simulink model "sampleModel7127_pp_difftest"  (R2018a)
settings: Solver=VariableStepAuto  StartTime=0.0  StopTime=10.0  RelTol=1e-3
undefined symbols (not defined in the file or in its folder): DiscIntNeverNeededParam, sigbuilder_block
libraries: simulink x258
(part 2 of 5)

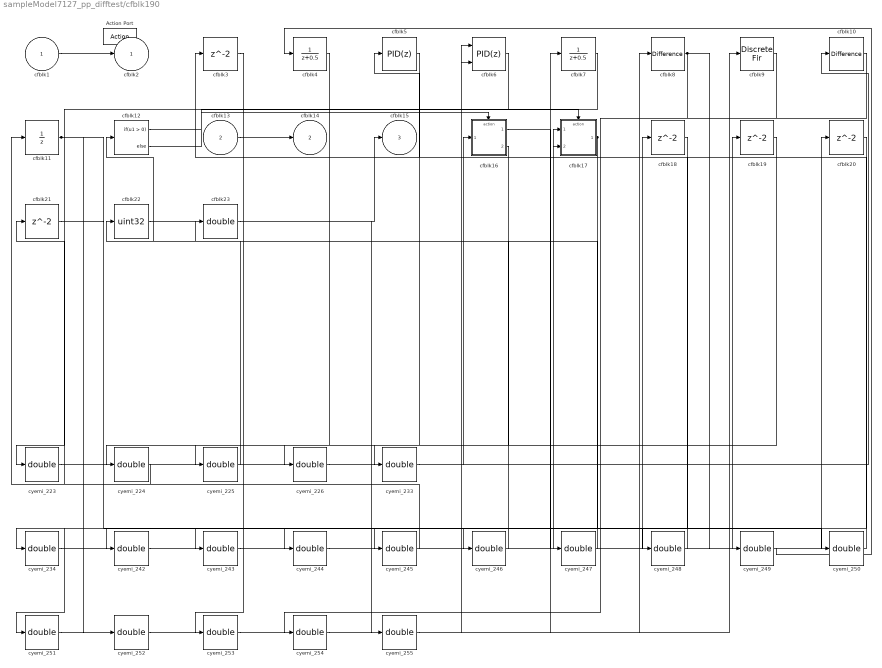
== system sampleModel7127_pp_difftest/cfblk190 ==
  cfblk1 : Inport
  cfblk13 : Inport  Port=2
  Action Port : ActionPort  ActionType=else
  cfblk10 : simulink/Discrete/Difference  ICPrevInput=0.0  OutMin=[]  OutMax=[]  OutDataTypeStr=double  OutputDataTypeScalingMode=double  OutDataType=fixdt(1, 16)  OutScaling=2^-10  DoSatur=off
  cfblk11 : UnitDelay  SampleTime=-1
  cfblk12 : If  SampleTime=1
  cfblk16 : Subsystem  TreatAsAtomicUnit=on
  cfblk17 : Subsystem  TreatAsAtomicUnit=on
  cfblk{3,18..21} (5 alike) : Delay
  cfblk22 : DataTypeConversion  OutDataTypeStr=uint32
  cfblk23 : DataTypeConversion  OutDataTypeStr=double
  cfblk4 : DiscreteTransferFcn
  cfblk5 : simulink/Continuous/PID Controller  Controller=PID  TimeDomain=Discrete-time  SampleTime=-1  IntegratorMethod=Forward Euler  FilterMethod=Forward Euler  Form=Parallel  UseFilter=on  ControllerParametersSource=internal  P=1  I=1  D=0  N=100  InitialConditionSource=internal  InitialConditionForIntegrator=0  InitialConditionForFilter=0  ExternalReset=none  LimitOutput=off  UpperSaturationLimit=inf  LowerSaturationLimit=-inf  LinearizeAsGain=off  AntiWindupMode=none  Kb=1  TrackingMode=off  Kt=1  PParamMin=[]  PParamMax=[]  IParamMin=[]  IParamMax=[]  DParamMin=[]  DParamMax=[]  NParamMin=[]  NParamMax=[]  KbParamMin=[]  KbParamMax=[]  KtParamMin=[]  KtParamMax=[]  POutMin=[]  POutMax=[]  IOutMin=[]  IOutMax=[]  DOutMin=[]  DOutMax=[]  NOutMin=[]  NOutMax=[]  KbOutMin=[]  KbOutMax=[]  KtOutMin=[]  KtOutMax=[]  IntegratorOutMin=[]  IntegratorOutMax=[]  FilterOutMin=[]  FilterOutMax=[]  SumOutMin=[]  SumOutMax=[]  SumI1OutMin=[]  SumI1OutMax=[]  SumI2OutMin=[]  SumI2OutMax=[]  SumI3OutMin=[]  SumI3OutMax=[]  SumDOutMin=[]  SumDOutMax=[]  SaturationOutMin=[]  SaturationOutMax=[]  IntegratorContinuousStateAttributes=''  IntegratorStateMustResolveToSignalObject=off  IntegratorRTWStateStorageClass=Auto  FilterContinuousStateAttributes=''  FilterStateMustResolveToSignalObject=off  FilterRTWStateStorageClass=Auto  DifferentiatorICPrevScaledInput=0  DifferentiatorOutMin=[]  DifferentiatorOutMax=[]  FilterDiffOutCoefMin=[]  FilterDiffOutCoefMax=[]  SumDenOutMin=[]  SumDenOutMax=[]  SumNumOutMin=[]  SumNumOutMax=[]  ReciprocalOutMin=[]  ReciprocalOutMax=[]  DivideOutMin=[]  DivideOutMax=[]  TunerSelectOption=Transfer Function Based (PID Tuner App)
  cfblk6 : simulink/Continuous/PID Controller (2DOF)  Controller=PID  TimeDomain=Discrete-time  SampleTime=-1  IntegratorMethod=Forward Euler  FilterMethod=Forward Euler  Form=Parallel  UseFilter=on  ControllerParametersSource=internal  P=1  I=1  D=0  N=100  b=1  c=1  InitialConditionSource=internal  InitialConditionForIntegrator=0  InitialConditionForFilter=0  ExternalReset=none  LimitOutput=off  UpperSaturationLimit=inf  LowerSaturationLimit=-inf  LinearizeAsGain=off  AntiWindupMode=none  Kb=1  TrackingMode=off  Kt=1  PParamMin=[]  PParamMax=[]  IParamMin=[]  IParamMax=[]  DParamMin=[]  DParamMax=[]  NParamMin=[]  NParamMax=[]  bParamMin=[]  bParamMax=[]  cParamMin=[]  cParamMax=[]  KbParamMin=[]  KbParamMax=[]  KtParamMin=[]  KtParamMax=[]  POutMin=[]  POutMax=[]  IOutMin=[]  IOutMax=[]  DOutMin=[]  DOutMax=[]  NOutMin=[]  NOutMax=[]  bOutMin=[]  bOutMax=[]  cOutMin=[]  cOutMax=[]  KbOutMin=[]  KbOutMax=[]  KtOutMin=[]  KtOutMax=[]  IntegratorOutMin=[]  IntegratorOutMax=[]  FilterOutMin=[]  FilterOutMax=[]  SumOutMin=[]  SumOutMax=[]  Sum1OutMin=[]  Sum1OutMax=[]  Sum2OutMin=[]  Sum2OutMax=[]  Sum3OutMin=[]  Sum3OutMax=[]  SumI1OutMin=[]  SumI1OutMax=[]  SumI2OutMin=[]  SumI2OutMax=[]  SumI3OutMin=[]  SumI3OutMax=[]  SumDOutMin=[]  SumDOutMax=[]  SaturationOutMin=[]  SaturationOutMax=[]  IntegratorContinuousStateAttributes=''  IntegratorStateMustResolveToSignalObject=off  IntegratorRTWStateStorageClass=Auto  FilterContinuousStateAttributes=''  FilterStateMustResolveToSignalObject=off  FilterRTWStateStorageClass=Auto  DifferentiatorICPrevScaledInput=0  DifferentiatorOutMin=[]  DifferentiatorOutMax=[]  FilterDiffOutCoefMin=[]  FilterDiffOutCoefMax=[]  SumDenOutMin=[]  SumDenOutMax=[]  SumNumOutMin=[]  SumNumOutMax=[]  ReciprocalOutMin=[]  ReciprocalOutMax=[]  DivideOutMin=[]  DivideOutMax=[]  TunerSelectOption=Transfer Function Based (PID Tuner App)
  cfblk7 : DiscreteTransferFcn
  cfblk8 : simulink/Discrete/Difference  ICPrevInput=0.0  OutMin=[]  OutMax=[]  OutDataTypeStr=double  OutputDataTypeScalingMode=double  OutDataType=fixdt(1, 16)  OutScaling=2^-10  DoSatur=off
  cfblk9 : DiscreteFir
  cyemi_{223..226,233..234,242..255} (20 alike) : DataTypeConversion  OutDataTypeStr=double
  cfblk2 : Outport
  cfblk14 : Outport  Port=2
  cfblk15 : Outport  Port=3
  wires:
  cfblk13/1 -> cfblk14/1
  cfblk1/1 -> cfblk2/1
  cfblk17/1(cfblk2) -> cyemi_242/1, cyemi_251/1
  cfblk8/1 -> cyemi_244/1, cyemi_249/1
  cfblk11/1 -> cyemi_245/1, cyemi_252/1
  cfblk12/1 -> cfblk16/Action
  cfblk12/2 -> cfblk17/Action
  cfblk22/1 -> cfblk15/1
  cyemi_223/1 -> cfblk10/1
  cfblk6/1 -> cyemi_223/1
  cyemi_224/1 -> cfblk11/1
  cfblk5/1 -> cyemi_224/1
  cyemi_225/1 -> cfblk12/1
  cfblk3/1 -> cyemi_225/1
  cyemi_226/1 -> cfblk16/1(cfblk1)
  cfblk19/1 -> cyemi_226/1
  cyemi_233/1 -> cfblk17/1(cfblk1)
  cfblk16/2(cfblk7) -> cyemi_233/1
  cyemi_234/1 -> cfblk17/2(cfblk9)
  cfblk20/1 -> cyemi_234/1
  cyemi_242/1 -> cfblk18/1
  cyemi_243/1 -> cfblk19/1
  cfblk7/1 -> cyemi_243/1
  cyemi_244/1 -> cfblk20/1
  cyemi_245/1 -> cfblk21/1
  cyemi_246/1 -> cfblk22/1
  cfblk9/1 -> cyemi_246/1
  cyemi_247/1 -> cfblk23/1
  cfblk16/1(cfblk2) -> cyemi_247/1
  cyemi_248/1 -> cfblk3/1
  cfblk18/1 -> cyemi_248/1
  cyemi_249/1 -> cfblk4/1
  cyemi_250/1 -> cfblk5/1
  cfblk21/1 -> cyemi_250/1
  cyemi_251/1 -> cfblk6/1
  cyemi_252/1 -> cfblk6/2
  cyemi_253/1 -> cfblk7/1
  cfblk4/1 -> cyemi_253/1
  cyemi_254/1 -> cfblk8/1
  cfblk10/1 -> cyemi_254/1
  cyemi_255/1 -> cfblk9/1
  cfblk23/1 -> cyemi_255/1

== system sampleModel7127_pp_difftest/cfblk191 ==
  cfblk1 : Inport
  Action Port : ActionPort  ActionType=then
  cfblk10 : DiscreteFir
  cfblk11 : simulink/Continuous/PID Controller  Controller=PID  TimeDomain=Discrete-time  SampleTime=-1  IntegratorMethod=Forward Euler  FilterMethod=Forward Euler  Form=Parallel  UseFilter=on  ControllerParametersSource=internal  P=1  I=1  D=0  N=100  InitialConditionSource=internal  InitialConditionForIntegrator=0  InitialConditionForFilter=0  ExternalReset=none  LimitOutput=off  UpperSaturationLimit=inf  LowerSaturationLimit=-inf  LinearizeAsGain=off  AntiWindupMode=none  Kb=1  TrackingMode=off  Kt=1  PParamMin=[]  PParamMax=[]  IParamMin=[]  IParamMax=[]  DParamMin=[]  DParamMax=[]  NParamMin=[]  NParamMax=[]  KbParamMin=[]  KbParamMax=[]  KtParamMin=[]  KtParamMax=[]  POutMin=[]  POutMax=[]  IOutMin=[]  IOutMax=[]  DOutMin=[]  DOutMax=[]  NOutMin=[]  NOutMax=[]  KbOutMin=[]  KbOutMax=[]  KtOutMin=[]  KtOutMax=[]  IntegratorOutMin=[]  IntegratorOutMax=[]  FilterOutMin=[]  FilterOutMax=[]  SumOutMin=[]  SumOutMax=[]  SumI1OutMin=[]  SumI1OutMax=[]  SumI2OutMin=[]  SumI2OutMax=[]  SumI3OutMin=[]  SumI3OutMax=[]  SumDOutMin=[]  SumDOutMax=[]  SaturationOutMin=[]  SaturationOutMax=[]  IntegratorContinuousStateAttributes=''  IntegratorStateMustResolveToSignalObject=off  IntegratorRTWStateStorageClass=Auto  FilterContinuousStateAttributes=''  FilterStateMustResolveToSignalObject=off  FilterRTWStateStorageClass=Auto  DifferentiatorICPrevScaledInput=0  DifferentiatorOutMin=[]  DifferentiatorOutMax=[]  FilterDiffOutCoefMin=[]  FilterDiffOutCoefMax=[]  SumDenOutMin=[]  SumDenOutMax=[]  SumNumOutMin=[]  SumNumOutMax=[]  ReciprocalOutMin=[]  ReciprocalOutMax=[]  DivideOutMin=[]  DivideOutMax=[]  TunerSelectOption=Transfer Function Based (PID Tuner App)
  cfblk12 : simulink/Continuous/PID Controller  Controller=PID  TimeDomain=Discrete-time  SampleTime=-1  IntegratorMethod=Forward Euler  FilterMethod=Forward Euler  Form=Parallel  UseFilter=on  ControllerParametersSource=internal  P=1  I=1  D=0  N=100  InitialConditionSource=internal  InitialConditionForIntegrator=0  InitialConditionForFilter=0  ExternalReset=none  LimitOutput=off  UpperSaturationLimit=inf  LowerSaturationLimit=-inf  LinearizeAsGain=off  AntiWindupMode=none  Kb=1  TrackingMode=off  Kt=1  PParamMin=[]  PParamMax=[]  IParamMin=[]  IParamMax=[]  DParamMin=[]  DParamMax=[]  NParamMin=[]  NParamMax=[]  KbParamMin=[]  KbParamMax=[]  KtParamMin=[]  KtParamMax=[]  POutMin=[]  POutMax=[]  IOutMin=[]  IOutMax=[]  DOutMin=[]  DOutMax=[]  NOutMin=[]  NOutMax=[]  KbOutMin=[]  KbOutMax=[]  KtOutMin=[]  KtOutMax=[]  IntegratorOutMin=[]  IntegratorOutMax=[]  FilterOutMin=[]  FilterOutMax=[]  SumOutMin=[]  SumOutMax=[]  SumI1OutMin=[]  SumI1OutMax=[]  SumI2OutMin=[]  SumI2OutMax=[]  SumI3OutMin=[]  SumI3OutMax=[]  SumDOutMin=[]  SumDOutMax=[]  SaturationOutMin=[]  SaturationOutMax=[]  IntegratorContinuousStateAttributes=''  IntegratorStateMustResolveToSignalObject=off  IntegratorRTWStateStorageClass=Auto  FilterContinuousStateAttributes=''  FilterStateMustResolveToSignalObject=off  FilterRTWStateStorageClass=Auto  DifferentiatorICPrevScaledInput=0  DifferentiatorOutMin=[]  DifferentiatorOutMax=[]  FilterDiffOutCoefMin=[]  FilterDiffOutCoefMax=[]  SumDenOutMin=[]  SumDenOutMax=[]  SumNumOutMin=[]  SumNumOutMax=[]  ReciprocalOutMin=[]  ReciprocalOutMax=[]  DivideOutMin=[]  DivideOutMax=[]  TunerSelectOption=Transfer Function Based (PID Tuner App)
  cfblk13 : simulink/Discrete/Difference  ICPrevInput=0.0  OutMin=[]  OutMax=[]  OutDataTypeStr=double  OutputDataTypeScalingMode=double  OutDataType=fixdt(1, 16)  OutScaling=2^-10  DoSatur=off
  cfblk14 : Delay
  cfblk15 : Delay
  cfblk3 : simulink/Discrete/Transfer Fcn First Order  PoleZ=0.95  ICPrevOutput=0.0  DoSatur=off
      settings: SourceProductName=Simulink
  cfblk4 : DiscreteZeroPole  Poles=[0 0.5]  Gain=1  SampleTime=-1
  cfblk5 : DiscreteTransferFcn
  cfblk6 : simulink/Continuous/PID Controller  Controller=PID  TimeDomain=Discrete-time  SampleTime=-1  IntegratorMethod=Forward Euler  FilterMethod=Forward Euler  Form=Parallel  UseFilter=on  ControllerParametersSource=internal  P=1  I=1  D=0  N=100  InitialConditionSource=internal  InitialConditionForIntegrator=0  InitialConditionForFilter=0  ExternalReset=none  LimitOutput=off  UpperSaturationLimit=inf  LowerSaturationLimit=-inf  LinearizeAsGain=off  AntiWindupMode=none  Kb=1  TrackingMode=off  Kt=1  PParamMin=[]  PParamMax=[]  IParamMin=[]  IParamMax=[]  DParamMin=[]  DParamMax=[]  NParamMin=[]  NParamMax=[]  KbParamMin=[]  KbParamMax=[]  KtParamMin=[]  KtParamMax=[]  POutMin=[]  POutMax=[]  IOutMin=[]  IOutMax=[]  DOutMin=[]  DOutMax=[]  NOutMin=[]  NOutMax=[]  KbOutMin=[]  KbOutMax=[]  KtOutMin=[]  KtOutMax=[]  IntegratorOutMin=[]  IntegratorOutMax=[]  FilterOutMin=[]  FilterOutMax=[]  SumOutMin=[]  SumOutMax=[]  SumI1OutMin=[]  SumI1OutMax=[]  SumI2OutMin=[]  SumI2OutMax=[]  SumI3OutMin=[]  SumI3OutMax=[]  SumDOutMin=[]  SumDOutMax=[]  SaturationOutMin=[]  SaturationOutMax=[]  IntegratorContinuousStateAttributes=''  IntegratorStateMustResolveToSignalObject=off  IntegratorRTWStateStorageClass=Auto  FilterContinuousStateAttributes=''  FilterStateMustResolveToSignalObject=off  FilterRTWStateStorageClass=Auto  DifferentiatorICPrevScaledInput=0  DifferentiatorOutMin=[]  DifferentiatorOutMax=[]  FilterDiffOutCoefMin=[]  FilterDiffOutCoefMax=[]  SumDenOutMin=[]  SumDenOutMax=[]  SumNumOutMin=[]  SumNumOutMax=[]  ReciprocalOutMin=[]  ReciprocalOutMax=[]  DivideOutMin=[]  DivideOutMax=[]  TunerSelectOption=Transfer Function Based (PID Tuner App)
  cfblk7 : simulink/Discrete/Transfer Fcn Real Zero  ZeroZ=0.75  ICPrevInput=0.0  DoSatur=off
      settings: SourceProductName=Simulink  SourceProductBaseCode=SL
  cfblk8 : simulink/Discrete/Tapped Delay  vinit=0.0  samptime=-1  NumDelays=1  DelayOrder=Oldest  includeCurrent=off
  cfblk9 : simulink/Discrete/Difference  ICPrevInput=0.0  OutMin=[]  OutMax=[]  OutDataTypeStr=double  OutputDataTypeScalingMode=double  OutDataType=fixdt(1, 16)  OutScaling=2^-10  DoSatur=off
  cyemi_{257..269} (13 alike) : DataTypeConversion  OutDataTypeStr=double
  cfblk2 : Outport
  wires:
  cfblk1/1 -> cfblk2/1
  cyemi_257/1 -> cfblk10/1
  cfblk11/1 -> cyemi_257/1
  cyemi_258/1 -> cfblk11/1
  cfblk7/1 -> cyemi_258/1
  cyemi_259/1 -> cfblk12/1
  cfblk3/1 -> cyemi_259/1
  cyemi_260/1 -> cfblk13/1
  cfblk8/1 -> cyemi_260/1
  cyemi_261/1 -> cfblk14/1
  cfblk10/1 -> cyemi_261/1
  cyemi_262/1 -> cfblk15/1
  cfblk9/1 -> cyemi_262/1
  cyemi_263/1 -> cfblk3/1
  cfblk14/1 -> cyemi_263/1
  cyemi_264/1 -> cfblk4/1
  cfblk15/1 -> cyemi_264/1
  cyemi_265/1 -> cfblk5/1
  cfblk13/1 -> cyemi_265/1
  cyemi_266/1 -> cfblk6/1
  cfblk5/1 -> cyemi_266/1
  cyemi_267/1 -> cfblk7/1
  cfblk6/1 -> cyemi_267/1
  cyemi_268/1 -> cfblk8/1
  cfblk12/1 -> cyemi_268/1
  cyemi_269/1 -> cfblk9/1
  cfblk4/1 -> cyemi_269/1

== system sampleModel7127_pp_difftest/cfblk192 ==
  cfblk1 : Inport
  cfblk8 : Inport  Port=2
  Action Port : ActionPort  ActionType=else
  cfblk3 : DiscreteStateSpace  SampleTime=-1
  cfblk4 : simulink/Discrete/Transfer Fcn Real Zero  ZeroZ=0.75  ICPrevInput=0.0  DoSatur=off
      settings: SourceProductName=Simulink  SourceProductBaseCode=SL
  cfblk5 : simulink/Discrete/Difference  ICPrevInput=0.0  OutMin=[]  OutMax=[]  OutDataTypeStr=double  OutputDataTypeScalingMode=double  OutDataType=fixdt(1, 16)  OutScaling=2^-10  DoSatur=off
  cfblk6 : DiscreteZeroPole  Poles=[0 0.5]  Gain=1  SampleTime=-1
  cfblk7 : simulink/Continuous/PID Controller (2DOF)  Controller=PID  TimeDomain=Discrete-time  SampleTime=-1  IntegratorMethod=Forward Euler  FilterMethod=Forward Euler  Form=Parallel  UseFilter=on  ControllerParametersSource=internal  P=1  I=1  D=0  N=100  b=1  c=1  InitialConditionSource=internal  InitialConditionForIntegrator=0  InitialConditionForFilter=0  ExternalReset=none  LimitOutput=off  UpperSaturationLimit=inf  LowerSaturationLimit=-inf  LinearizeAsGain=off  AntiWindupMode=none  Kb=1  TrackingMode=off  Kt=1  PParamMin=[]  PParamMax=[]  IParamMin=[]  IParamMax=[]  DParamMin=[]  DParamMax=[]  NParamMin=[]  NParamMax=[]  bParamMin=[]  bParamMax=[]  cParamMin=[]  cParamMax=[]  KbParamMin=[]  KbParamMax=[]  KtParamMin=[]  KtParamMax=[]  POutMin=[]  POutMax=[]  IOutMin=[]  IOutMax=[]  DOutMin=[]  DOutMax=[]  NOutMin=[]  NOutMax=[]  bOutMin=[]  bOutMax=[]  cOutMin=[]  cOutMax=[]  KbOutMin=[]  KbOutMax=[]  KtOutMin=[]  KtOutMax=[]  IntegratorOutMin=[]  IntegratorOutMax=[]  FilterOutMin=[]  FilterOutMax=[]  SumOutMin=[]  SumOutMax=[]  Sum1OutMin=[]  Sum1OutMax=[]  Sum2OutMin=[]  Sum2OutMax=[]  Sum3OutMin=[]  Sum3OutMax=[]  SumI1OutMin=[]  SumI1OutMax=[]  SumI2OutMin=[]  SumI2OutMax=[]  SumI3OutMin=[]  SumI3OutMax=[]  SumDOutMin=[]  SumDOutMax=[]  SaturationOutMin=[]  SaturationOutMax=[]  IntegratorContinuousStateAttributes=''  IntegratorStateMustResolveToSignalObject=off  IntegratorRTWStateStorageClass=Auto  FilterContinuousStateAttributes=''  FilterStateMustResolveToSignalObject=off  FilterRTWStateStorageClass=Auto  DifferentiatorICPrevScaledInput=0  DifferentiatorOutMin=[]  DifferentiatorOutMax=[]  FilterDiffOutCoefMin=[]  FilterDiffOutCoefMax=[]  SumDenOutMin=[]  SumDenOutMax=[]  SumNumOutMin=[]  SumNumOutMax=[]  ReciprocalOutMin=[]  ReciprocalOutMax=[]  DivideOutMin=[]  DivideOutMax=[]  TunerSelectOption=Transfer Function Based (PID Tuner App)
  cfblk9 : Delay
  cyemi_{272..278} (7 alike) : DataTypeConversion  OutDataTypeStr=double
  cfblk2 : Outport
  wires:
  cfblk1/1 -> cfblk2/1
  cyemi_272/1 -> cfblk3/1
  cfblk9/1 -> cyemi_272/1
  cyemi_273/1 -> cfblk4/1
  cfblk5/1 -> cyemi_273/1
  cyemi_274/1 -> cfblk5/1
  cfblk7/1 -> cyemi_274/1
  cyemi_275/1 -> cfblk6/1
  cfblk4/1 -> cyemi_275/1
  cyemi_276/1 -> cfblk7/1
  cfblk8/1 -> cyemi_276/1
  cyemi_277/1 -> cfblk7/2
  cfblk3/1 -> cyemi_277/1
  cyemi_278/1 -> cfblk9/1
  cfblk6/1 -> cyemi_278/1

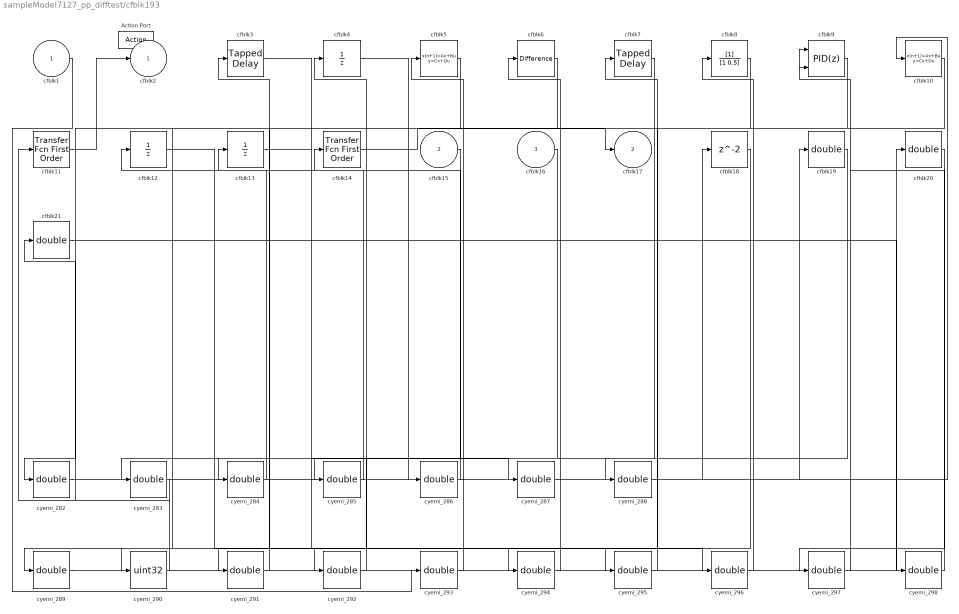
== system sampleModel7127_pp_difftest/cfblk193 ==
  cfblk1 : Inport
  cfblk15 : Inport  Port=2
  cfblk16 : Inport  Port=3
  Action Port : ActionPort  ActionType=then
  cfblk10 : DiscreteStateSpace  SampleTime=-1
  cfblk11 : simulink/Discrete/Transfer Fcn First Order  PoleZ=0.95  ICPrevOutput=0.0  DoSatur=off
      settings: SourceProductName=Simulink
  cfblk12 : UnitDelay  SampleTime=-1
  cfblk13 : UnitDelay  SampleTime=-1
  cfblk14 : simulink/Discrete/Transfer Fcn First Order  PoleZ=0.95  ICPrevOutput=0.0  DoSatur=off
      settings: SourceProductName=Simulink
  cfblk18 : Delay
  cfblk19 : DataTypeConversion  OutDataTypeStr=double
  cfblk20 : DataTypeConversion  OutDataTypeStr=double
  cfblk21 : DataTypeConversion  OutDataTypeStr=double
  cfblk3 : simulink/Discrete/Tapped Delay  vinit=0.0  samptime=-1  NumDelays=1  DelayOrder=Oldest  includeCurrent=off
  cfblk4 : UnitDelay  SampleTime=-1
  cfblk5 : DiscreteStateSpace  SampleTime=-1
  cfblk6 : simulink/Discrete/Difference  ICPrevInput=0.0  OutMin=[]  OutMax=[]  OutDataTypeStr=double  OutputDataTypeScalingMode=double  OutDataType=fixdt(1, 16)  OutScaling=2^-10  DoSatur=off
  cfblk7 : simulink/Discrete/Tapped Delay  vinit=0.0  samptime=-1  NumDelays=1  DelayOrder=Oldest  includeCurrent=off
  cfblk8 : DiscreteFilter
  cfblk9 : simulink/Continuous/PID Controller (2DOF)  Controller=PID  TimeDomain=Discrete-time  SampleTime=-1  IntegratorMethod=Forward Euler  FilterMethod=Forward Euler  Form=Parallel  UseFilter=on  ControllerParametersSource=internal  P=1  I=1  D=0  N=100  b=1  c=1  InitialConditionSource=internal  InitialConditionForIntegrator=0  InitialConditionForFilter=0  ExternalReset=none  LimitOutput=off  UpperSaturationLimit=inf  LowerSaturationLimit=-inf  LinearizeAsGain=off  AntiWindupMode=none  Kb=1  TrackingMode=off  Kt=1  PParamMin=[]  PParamMax=[]  IParamMin=[]  IParamMax=[]  DParamMin=[]  DParamMax=[]  NParamMin=[]  NParamMax=[]  bParamMin=[]  bParamMax=[]  cParamMin=[]  cParamMax=[]  KbParamMin=[]  KbParamMax=[]  KtParamMin=[]  KtParamMax=[]  POutMin=[]  POutMax=[]  IOutMin=[]  IOutMax=[]  DOutMin=[]  DOutMax=[]  NOutMin=[]  NOutMax=[]  bOutMin=[]  bOutMax=[]  cOutMin=[]  cOutMax=[]  KbOutMin=[]  KbOutMax=[]  KtOutMin=[]  KtOutMax=[]  IntegratorOutMin=[]  IntegratorOutMax=[]  FilterOutMin=[]  FilterOutMax=[]  SumOutMin=[]  SumOutMax=[]  Sum1OutMin=[]  Sum1OutMax=[]  Sum2OutMin=[]  Sum2OutMax=[]  Sum3OutMin=[]  Sum3OutMax=[]  SumI1OutMin=[]  SumI1OutMax=[]  SumI2OutMin=[]  SumI2OutMax=[]  SumI3OutMin=[]  SumI3OutMax=[]  SumDOutMin=[]  SumDOutMax=[]  SaturationOutMin=[]  SaturationOutMax=[]  IntegratorContinuousStateAttributes=''  IntegratorStateMustResolveToSignalObject=off  IntegratorRTWStateStorageClass=Auto  FilterContinuousStateAttributes=''  FilterStateMustResolveToSignalObject=off  FilterRTWStateStorageClass=Auto  DifferentiatorICPrevScaledInput=0  DifferentiatorOutMin=[]  DifferentiatorOutMax=[]  FilterDiffOutCoefMin=[]  FilterDiffOutCoefMax=[]  SumDenOutMin=[]  SumDenOutMax=[]  SumNumOutMin=[]  SumNumOutMax=[]  ReciprocalOutMin=[]  ReciprocalOutMax=[]  DivideOutMin=[]  DivideOutMax=[]  TunerSelectOption=Transfer Function Based (PID Tuner App)
  cyemi_{282..289,291..298} (16 alike) : DataTypeConversion  OutDataTypeStr=double
  cyemi_290 : DataTypeConversion  OutDataTypeStr=uint32
  cfblk2 : Outport
  cfblk17 : Outport  Port=2
  wires:
  cfblk14/1 -> cfblk17/1
  cfblk11/1 -> cfblk2/1
  cyemi_282/1 -> cfblk10/1
  cfblk5/1 -> cyemi_282/1
  cyemi_283/1 -> cfblk11/1
  cfblk6/1 -> cyemi_283/1
  cyemi_284/1 -> cfblk12/1
  cfblk15/1 -> cyemi_284/1
  cyemi_285/1 -> cfblk13/1
  cfblk19/1 -> cyemi_285/1
  cyemi_286/1 -> cfblk14/1
  cfblk4/1 -> cyemi_286/1
  cyemi_287/1 -> cfblk18/1
  cfblk13/1 -> cyemi_287/1
  cyemi_288/1 -> cfblk19/1
  cfblk9/1 -> cyemi_288/1
  cyemi_289/1 -> cfblk20/1
  cfblk18/1 -> cyemi_289/1
  cyemi_290/1 -> cfblk21/1
  cfblk16/1 -> cyemi_290/1
  cyemi_291/1 -> cfblk3/1
  cfblk8/1 -> cyemi_291/1
  cyemi_292/1 -> cfblk4/1
  cfblk7/1 -> cyemi_292/1
  cyemi_293/1 -> cfblk5/1
  cfblk1/1 -> cyemi_293/1
  cyemi_294/1 -> cfblk6/1
  cfblk3/1 -> cyemi_294/1
  cyemi_295/1 -> cfblk7/1
  cfblk10/1 -> cyemi_295/1
  cyemi_296/1 -> cfblk8/1
  cfblk12/1 -> cyemi_296/1
  cyemi_297/1 -> cfblk9/1
  cfblk20/1 -> cyemi_297/1
  cyemi_298/1 -> cfblk9/2
  cfblk21/1 -> cyemi_298/1

== system sampleModel7127_pp_difftest/cfblk194 ==
  cfblk1 : Inport
  cfblk6 : Inport  Port=2
  cfblk7 : Inport  Port=3
  cfblk8 : Inport  Port=4
  Action Port : ActionPort  ActionType=else
  cfblk10 : Subsystem  TreatAsAtomicUnit=on
  cfblk11 : Subsystem  TreatAsAtomicUnit=on
  cfblk12 : Delay
  cfblk3 : simulink/Discrete/Transfer Fcn Lead or Lag  PoleZ=0.95  ZeroZ=0.75  ICPrevOutput=0.0  ICPrevInput=0.0  DoSatur=off
      settings: SourceProductName=Simulink  SourceProductBaseCode=SL
  cfblk4 : Delay
  cfblk5 : If  SampleTime=1
  cyemi_{303..304,314..315,325..328} (8 alike) : DataTypeConversion  OutDataTypeStr=double
  cfblk2 : Outport
  cfblk9 : Outport  Port=2
  wires:
  cfblk10/2(cfblk11) -> cfblk2/1
  cfblk11/1(cfblk2) -> cfblk9/1
  cfblk5/1 -> cfblk10/Action
  cfblk5/2 -> cfblk11/Action
  cyemi_303/1 -> cfblk10/1(cfblk1)
  cfblk3/1 -> cyemi_303/1
  cyemi_304/1 -> cfblk10/2(cfblk10)
  cfblk6/1 -> cyemi_304/1
  cyemi_314/1 -> cfblk11/1(cfblk1)
  cfblk4/1 -> cyemi_314/1
  cyemi_315/1 -> cfblk11/2(cfblk10)
  cfblk8/1 -> cyemi_315/1
  cyemi_325/1 -> cfblk12/1
  cfblk10/1(cfblk2) -> cyemi_325/1
  cyemi_326/1 -> cfblk3/1
  cfblk12/1 -> cyemi_326/1
  cyemi_327/1 -> cfblk4/1
  cfblk1/1 -> cyemi_327/1
  cyemi_328/1 -> cfblk5/1
  cfblk7/1 -> cyemi_328/1

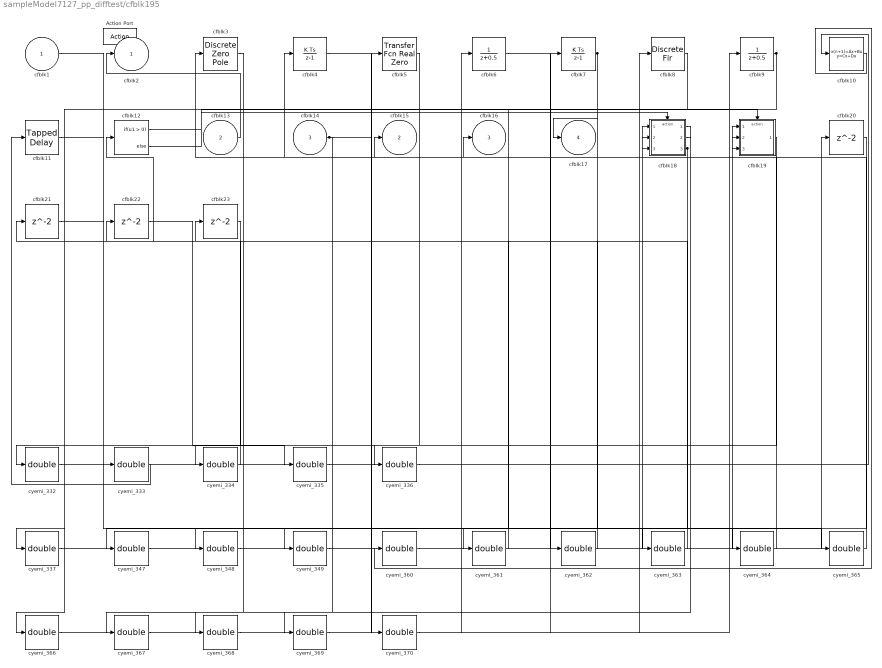
== system sampleModel7127_pp_difftest/cfblk195 ==
  cfblk1 : Inport
  cfblk13 : Inport  Port=2
  cfblk14 : Inport  Port=3
  Action Port : ActionPort  ActionType=then
  cfblk10 : DiscreteStateSpace  SampleTime=-1
  cfblk11 : simulink/Discrete/Tapped Delay  vinit=0.0  samptime=-1  NumDelays=1  DelayOrder=Oldest  includeCurrent=off
  cfblk12 : If  SampleTime=1
  cfblk18 : Subsystem  TreatAsAtomicUnit=on
  cfblk19 : Subsystem  TreatAsAtomicUnit=on
  cfblk{20..23} (4 alike) : Delay
  cfblk3 : DiscreteZeroPole  Poles=[0 0.5]  Gain=1  SampleTime=-1
  cfblk4 : DiscreteIntegrator  SampleTime=-1  OutDataTypeStr=double  ICPrevOutput=DiscIntNeverNeededParam  ICPrevScaledInput=DiscIntNeverNeededParam
  cfblk5 : simulink/Discrete/Transfer Fcn Real Zero  ZeroZ=0.75  ICPrevInput=0.0  DoSatur=off
      settings: SourceProductName=Simulink  SourceProductBaseCode=SL
  cfblk6 : DiscreteTransferFcn
  cfblk7 : DiscreteIntegrator  SampleTime=-1  OutDataTypeStr=double  ICPrevOutput=DiscIntNeverNeededParam  ICPrevScaledInput=DiscIntNeverNeededParam
  cfblk8 : DiscreteFir
  cfblk9 : DiscreteTransferFcn
  cyemi_{332..337,347..349,360..370} (20 alike) : DataTypeConversion  OutDataTypeStr=double
  cfblk2 : Outport
  cfblk15 : Outport  Port=2
  cfblk16 : Outport  Port=3
  cfblk17 : Outport  Port=4
  wires:
  cfblk9/1 -> cyemi_337/1, cyemi_361/1
  cfblk13/1 -> cfblk2/1
  cfblk7/1 -> cfblk17/1, cyemi_349/1
  cfblk18/2(cfblk13) -> cfblk16/1
  cfblk18/3(cfblk14) -> cfblk15/1, cyemi_363/1
  cfblk14/1 -> cyemi_364/1, cyemi_369/1
  cfblk12/1 -> cfblk18/Action
  cfblk12/2 -> cfblk19/Action
  cyemi_332/1 -> cfblk10/1
  cfblk19/1(cfblk2) -> cyemi_332/1
  cyemi_333/1 -> cfblk11/1
  cfblk1/1 -> cyemi_333/1
  cyemi_334/1 -> cfblk12/1
  cfblk23/1 -> cyemi_334/1
  cyemi_335/1 -> cfblk18/1(cfblk1)
  cfblk22/1 -> cyemi_335/1
  cyemi_336/1 -> cfblk18/2(cfblk11)
  cfblk5/1 -> cyemi_336/1
  cyemi_337/1 -> cfblk18/3(cfblk12)
  cyemi_347/1 -> cfblk19/1(cfblk1)
  cfblk20/1 -> cyemi_347/1
  cyemi_348/1 -> cfblk19/2(cfblk11)
  cfblk11/1 -> cyemi_348/1
  cyemi_349/1 -> cfblk19/3(cfblk12)
  cyemi_360/1 -> cfblk20/1
  cfblk10/1 -> cyemi_360/1
  cyemi_361/1 -> cfblk21/1
  cyemi_362/1 -> cfblk22/1
  cfblk6/1 -> cyemi_362/1
  cyemi_363/1 -> cfblk23/1
  cyemi_364/1 -> cfblk3/1
  cyemi_365/1 -> cfblk4/1
  cfblk21/1 -> cyemi_365/1
  cyemi_366/1 -> cfblk5/1
  cfblk8/1 -> cyemi_366/1
  cyemi_367/1 -> cfblk6/1
  cfblk18/1(cfblk2) -> cyemi_367/1
  cyemi_368/1 -> cfblk7/1
  cfblk3/1 -> cyemi_368/1
  cyemi_369/1 -> cfblk8/1
  cyemi_370/1 -> cfblk9/1
  cfblk4/1 -> cyemi_370/1

== system sampleModel7127_pp_difftest/cfblk196 ==
  cfblk1 : Inport
  Action Port : ActionPort  ActionType=else
  cfblk3 : Delay  ShowEnablePort=on
      settings: InputPortMap=u0,e6
  cfblk4 : UnitDelay  SampleTime=-1
  cfblk5 : simulink/Continuous/PID Controller (2DOF)  Controller=PID  TimeDomain=Discrete-time  SampleTime=-1  IntegratorMethod=Forward Euler  FilterMethod=Forward Euler  Form=Parallel  UseFilter=on  ControllerParametersSource=internal  P=1  I=1  D=0  N=100  b=1  c=1  InitialConditionSource=internal  InitialConditionForIntegrator=0  InitialConditionForFilter=0  ExternalReset=none  LimitOutput=off  UpperSaturationLimit=inf  LowerSaturationLimit=-inf  LinearizeAsGain=off  AntiWindupMode=none  Kb=1  TrackingMode=off  Kt=1  PParamMin=[]  PParamMax=[]  IParamMin=[]  IParamMax=[]  DParamMin=[]  DParamMax=[]  NParamMin=[]  NParamMax=[]  bParamMin=[]  bParamMax=[]  cParamMin=[]  cParamMax=[]  KbParamMin=[]  KbParamMax=[]  KtParamMin=[]  KtParamMax=[]  POutMin=[]  POutMax=[]  IOutMin=[]  IOutMax=[]  DOutMin=[]  DOutMax=[]  NOutMin=[]  NOutMax=[]  bOutMin=[]  bOutMax=[]  cOutMin=[]  cOutMax=[]  KbOutMin=[]  KbOutMax=[]  KtOutMin=[]  KtOutMax=[]  IntegratorOutMin=[]  IntegratorOutMax=[]  FilterOutMin=[]  FilterOutMax=[]  SumOutMin=[]  SumOutMax=[]  Sum1OutMin=[]  Sum1OutMax=[]  Sum2OutMin=[]  Sum2OutMax=[]  Sum3OutMin=[]  Sum3OutMax=[]  SumI1OutMin=[]  SumI1OutMax=[]  SumI2OutMin=[]  SumI2OutMax=[]  SumI3OutMin=[]  SumI3OutMax=[]  SumDOutMin=[]  SumDOutMax=[]  SaturationOutMin=[]  SaturationOutMax=[]  IntegratorContinuousStateAttributes=''  IntegratorStateMustResolveToSignalObject=off  IntegratorRTWStateStorageClass=Auto  FilterContinuousStateAttributes=''  FilterStateMustResolveToSignalObject=off  FilterRTWStateStorageClass=Auto  DifferentiatorICPrevScaledInput=0  DifferentiatorOutMin=[]  DifferentiatorOutMax=[]  FilterDiffOutCoefMin=[]  FilterDiffOutCoefMax=[]  SumDenOutMin=[]  SumDenOutMax=[]  SumNumOutMin=[]  SumNumOutMax=[]  ReciprocalOutMin=[]  ReciprocalOutMax=[]  DivideOutMin=[]  DivideOutMax=[]  TunerSelectOption=Transfer Function Based (PID Tuner App)
  cfblk6 : simulink/Discrete/Tapped Delay  vinit=0.0  samptime=-1  NumDelays=1  DelayOrder=Oldest  includeCurrent=off
  cfblk7 : DiscreteStateSpace  SampleTime=-1
  cfblk8 : DiscreteFilter
  cfblk9 : Delay  ShowEnablePort=on
      settings: InputPortMap=u0,e6
  cyemi_{372..381} (10 alike) : DataTypeConversion  OutDataTypeStr=double
  cfblk2 : Outport
  cfblk10 : Outport  Port=2
  wires:
  cfblk4/1 -> cyemi_377/1, cyemi_378/1
  cfblk3/1 -> cfblk10/1
  cfblk9/1 -> cfblk2/1
  cyemi_372/1 -> cfblk3/1
  cfblk7/1 -> cyemi_372/1, cyemi_373/1
  cyemi_373/1 -> cfblk3/2
  cyemi_374/1 -> cfblk4/1
  cfblk5/1 -> cyemi_374/1
  cyemi_375/1 -> cfblk5/1
  cfblk8/1 -> cyemi_375/1, cyemi_376/1
  cyemi_376/1 -> cfblk5/2
  cyemi_377/1 -> cfblk6/1
  cyemi_378/1 -> cfblk7/1
  cyemi_379/1 -> cfblk8/1
  cfblk1/1 -> cyemi_379/1
  cyemi_380/1 -> cfblk9/1
  cfblk6/1 -> cyemi_380/1, cyemi_381/1
  cyemi_381/1 -> cfblk9/2

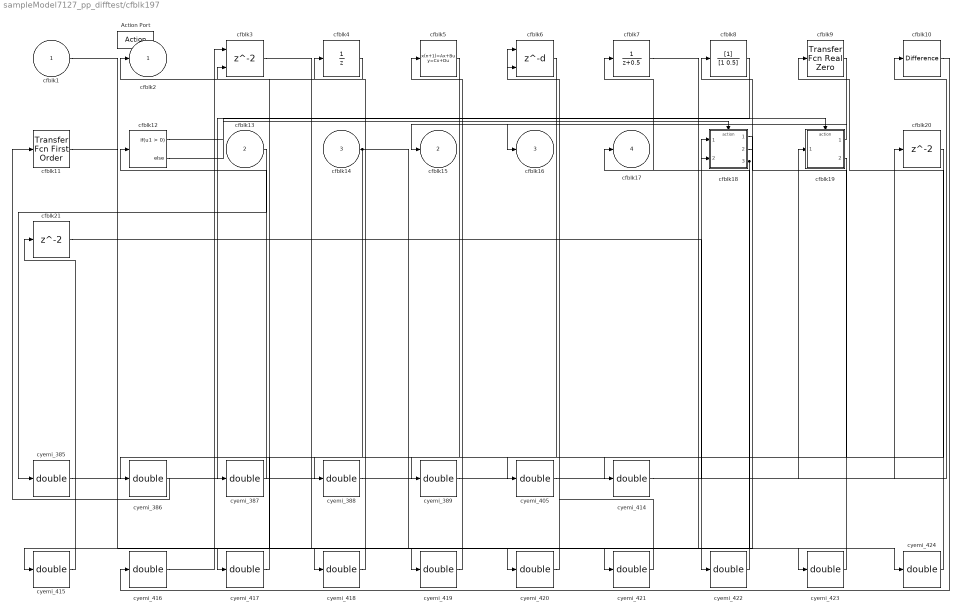
== system sampleModel7127_pp_difftest/cfblk197 ==
  cfblk1 : Inport
  cfblk13 : Inport  Port=2
  cfblk14 : Inport  Port=3
  Action Port : ActionPort  ActionType=then
  cfblk10 : simulink/Discrete/Difference  ICPrevInput=0.0  OutMin=[]  OutMax=[]  OutDataTypeStr=double  OutputDataTypeScalingMode=double  OutDataType=fixdt(1, 16)  OutScaling=2^-10  DoSatur=off
  cfblk11 : simulink/Discrete/Transfer Fcn First Order  PoleZ=0.95  ICPrevOutput=0.0  DoSatur=off
      settings: SourceProductName=Simulink
  cfblk12 : If  SampleTime=1
  cfblk18 : Subsystem  TreatAsAtomicUnit=on
  cfblk19 : Subsystem  TreatAsAtomicUnit=on
  cfblk20 : Delay
  cfblk21 : Delay
  cfblk3 : Delay  ShowEnablePort=on
      settings: InputPortMap=u0,e6
  cfblk4 : UnitDelay  SampleTime=-1
  cfblk5 : DiscreteStateSpace  SampleTime=-1
  cfblk6 : Delay  DelayLengthSource=Input port
      settings: InputPortMap=u0,p1
  cfblk7 : DiscreteTransferFcn
  cfblk8 : DiscreteFilter
  cfblk9 : simulink/Discrete/Transfer Fcn Real Zero  ZeroZ=0.75  ICPrevInput=0.0  DoSatur=off
      settings: SourceProductName=Simulink  SourceProductBaseCode=SL
  cyemi_{385..389,405,414..424} (17 alike) : DataTypeConversion  OutDataTypeStr=double
  cfblk2 : Outport
  cfblk15 : Outport  Port=2
  cfblk16 : Outport  Port=3
  cfblk17 : Outport  Port=4
  wires:
  cfblk4/1 -> cfblk2/1
  cfblk9/1 -> cfblk16/1
  cfblk19/1(cfblk2) -> cfblk15/1
  cfblk18/3(cfblk14) -> cfblk17/1, cyemi_415/1
  cfblk14/1 -> cyemi_388/1, cyemi_421/1
  cfblk12/1 -> cfblk18/Action
  cfblk12/2 -> cfblk19/Action
  cyemi_385/1 -> cfblk10/1
  cfblk13/1 -> cyemi_385/1
  cyemi_386/1 -> cfblk11/1
  cfblk5/1 -> cyemi_386/1
  cyemi_387/1 -> cfblk12/1
  cfblk8/1 -> cyemi_387/1
  cyemi_388/1 -> cfblk18/1(cfblk1)
  cyemi_389/1 -> cfblk18/2(cfblk12)
  cfblk20/1 -> cyemi_389/1
  cyemi_405/1 -> cfblk19/1(cfblk1)
  cfblk18/2(cfblk13) -> cyemi_405/1
  cyemi_414/1 -> cfblk20/1
  cfblk19/2(cfblk8) -> cyemi_414/1
  cyemi_415/1 -> cfblk21/1
  cyemi_416/1 -> cfblk3/1
  cfblk10/1 -> cyemi_416/1
  cyemi_417/1 -> cfblk3/2
  cfblk6/1 -> cyemi_417/1
  cyemi_418/1 -> cfblk4/1
  cfblk11/1 -> cyemi_418/1
  cyemi_419/1 -> cfblk5/1
  cfblk18/1(cfblk2) -> cyemi_419/1
  cyemi_420/1 -> cfblk6/1
  cfblk1/1 -> cyemi_420/1
  cyemi_421/1 -> cfblk6/2
  cyemi_422/1 -> cfblk7/1
  cfblk21/1 -> cyemi_422/1
  cyemi_423/1 -> cfblk8/1
  cfblk7/1 -> cyemi_423/1
  cyemi_424/1 -> cfblk9/1
  cfblk3/1 -> cyemi_424/1

== system sampleModel7127_pp_difftest/cfblk198 ==
  cfblk1 : Inport
  Action Port : ActionPort  ActionType=else
  cfblk3 : Delay  ShowEnablePort=on
      settings: InputPortMap=u0,e6
  cfblk4 : simulink/Discrete/Difference  ICPrevInput=0.0  OutMin=[]  OutMax=[]  OutDataTypeStr=double  OutputDataTypeScalingMode=double  OutDataType=fixdt(1, 16)  OutScaling=2^-10  DoSatur=off
  cfblk5 : UnitDelay  SampleTime=-1
  cfblk6 : simulink/Continuous/PID Controller  Controller=PID  TimeDomain=Discrete-time  SampleTime=-1  IntegratorMethod=Forward Euler  FilterMethod=Forward Euler  Form=Parallel  UseFilter=on  ControllerParametersSource=internal  P=1  I=1  D=0  N=100  InitialConditionSource=internal  InitialConditionForIntegrator=0  InitialConditionForFilter=0  ExternalReset=none  LimitOutput=off  UpperSaturationLimit=inf  LowerSaturationLimit=-inf  LinearizeAsGain=off  AntiWindupMode=none  Kb=1  TrackingMode=off  Kt=1  PParamMin=[]  PParamMax=[]  IParamMin=[]  IParamMax=[]  DParamMin=[]  DParamMax=[]  NParamMin=[]  NParamMax=[]  KbParamMin=[]  KbParamMax=[]  KtParamMin=[]  KtParamMax=[]  POutMin=[]  POutMax=[]  IOutMin=[]  IOutMax=[]  DOutMin=[]  DOutMax=[]  NOutMin=[]  NOutMax=[]  KbOutMin=[]  KbOutMax=[]  KtOutMin=[]  KtOutMax=[]  IntegratorOutMin=[]  IntegratorOutMax=[]  FilterOutMin=[]  FilterOutMax=[]  SumOutMin=[]  SumOutMax=[]  SumI1OutMin=[]  SumI1OutMax=[]  SumI2OutMin=[]  SumI2OutMax=[]  SumI3OutMin=[]  SumI3OutMax=[]  SumDOutMin=[]  SumDOutMax=[]  SaturationOutMin=[]  SaturationOutMax=[]  IntegratorContinuousStateAttributes=''  IntegratorStateMustResolveToSignalObject=off  IntegratorRTWStateStorageClass=Auto  FilterContinuousStateAttributes=''  FilterStateMustResolveToSignalObject=off  FilterRTWStateStorageClass=Auto  DifferentiatorICPrevScaledInput=0  DifferentiatorOutMin=[]  DifferentiatorOutMax=[]  FilterDiffOutCoefMin=[]  FilterDiffOutCoefMax=[]  SumDenOutMin=[]  SumDenOutMax=[]  SumNumOutMin=[]  SumNumOutMax=[]  ReciprocalOutMin=[]  ReciprocalOutMax=[]  DivideOutMin=[]  DivideOutMax=[]  TunerSelectOption=Transfer Function Based (PID Tuner App)
  cfblk7 : Delay  ShowEnablePort=on
      settings: InputPortMap=u0,e6
  cfblk8 : simulink/Continuous/PID Controller  Controller=PID  TimeDomain=Discrete-time  SampleTime=-1  IntegratorMethod=Forward Euler  FilterMethod=Forward Euler  Form=Parallel  UseFilter=on  ControllerParametersSource=internal  P=1  I=1  D=0  N=100  InitialConditionSource=internal  InitialConditionForIntegrator=0  InitialConditionForFilter=0  ExternalReset=none  LimitOutput=off  UpperSaturationLimit=inf  LowerSaturationLimit=-inf  LinearizeAsGain=off  AntiWindupMode=none  Kb=1  TrackingMode=off  Kt=1  PParamMin=[]  PParamMax=[]  IParamMin=[]  IParamMax=[]  DParamMin=[]  DParamMax=[]  NParamMin=[]  NParamMax=[]  KbParamMin=[]  KbParamMax=[]  KtParamMin=[]  KtParamMax=[]  POutMin=[]  POutMax=[]  IOutMin=[]  IOutMax=[]  DOutMin=[]  DOutMax=[]  NOutMin=[]  NOutMax=[]  KbOutMin=[]  KbOutMax=[]  KtOutMin=[]  KtOutMax=[]  IntegratorOutMin=[]  IntegratorOutMax=[]  FilterOutMin=[]  FilterOutMax=[]  SumOutMin=[]  SumOutMax=[]  SumI1OutMin=[]  SumI1OutMax=[]  SumI2OutMin=[]  SumI2OutMax=[]  SumI3OutMin=[]  SumI3OutMax=[]  SumDOutMin=[]  SumDOutMax=[]  SaturationOutMin=[]  SaturationOutMax=[]  IntegratorContinuousStateAttributes=''  IntegratorStateMustResolveToSignalObject=off  IntegratorRTWStateStorageClass=Auto  FilterContinuousStateAttributes=''  FilterStateMustResolveToSignalObject=off  FilterRTWStateStorageClass=Auto  DifferentiatorICPrevScaledInput=0  DifferentiatorOutMin=[]  DifferentiatorOutMax=[]  FilterDiffOutCoefMin=[]  FilterDiffOutCoefMax=[]  SumDenOutMin=[]  SumDenOutMax=[]  SumNumOutMin=[]  SumNumOutMax=[]  ReciprocalOutMin=[]  ReciprocalOutMax=[]  DivideOutMin=[]  DivideOutMax=[]  TunerSelectOption=Transfer Function Based (PID Tuner App)
  cfblk9 : simulink/Discrete/Tapped Delay  vinit=0.0  samptime=-1  NumDelays=1  DelayOrder=Oldest  includeCurrent=off
  cyemi_{426..434} (9 alike) : DataTypeConversion  OutDataTypeStr=double
  cfblk2 : Outport
  cfblk10 : Outport  Port=2
  wires:
  cfblk7/1 -> cfblk2/1
  cfblk5/1 -> cyemi_427/1, cyemi_430/1, cyemi_433/1
  cfblk1/1 -> cfblk10/1, cyemi_429/1
  cyemi_426/1 -> cfblk3/1
  cfblk6/1 -> cyemi_426/1
  cyemi_427/1 -> cfblk3/2
  cyemi_428/1 -> cfblk4/1
  cfblk9/1 -> cyemi_428/1
  cyemi_429/1 -> cfblk5/1
  cyemi_430/1 -> cfblk6/1
  cyemi_431/1 -> cfblk7/1
  cfblk4/1 -> cyemi_431/1
  cyemi_432/1 -> cfblk7/2
  cfblk3/1 -> cyemi_432/1
  cyemi_433/1 -> cfblk8/1
  cyemi_434/1 -> cfblk9/1
  cfblk8/1 -> cyemi_434/1

== system sampleModel7127_pp_difftest/cfblk199 ==
  cfblk1 : Inport
  Action Port : ActionPort  ActionType=then
  cfblk11 : Delay
  cfblk3 : simulink/Discrete/Transfer Fcn Lead or Lag  PoleZ=0.95  ZeroZ=0.75  ICPrevOutput=0.0  ICPrevInput=0.0  DoSatur=off
      settings: SourceProductName=Simulink  SourceProductBaseCode=SL
  cfblk4 : DiscreteStateSpace  SampleTime=-1
  cfblk5 : simulink/Discrete/Transfer Fcn First Order  PoleZ=0.95  ICPrevOutput=0.0  DoSatur=off
      settings: SourceProductName=Simulink
  cfblk6 : Delay  DelayLengthSource=Input port
      settings: InputPortMap=u0,p1
  cfblk7 : simulink/Discrete/Transfer Fcn First Order  PoleZ=0.95  ICPrevOutput=0.0  DoSatur=off
      settings: SourceProductName=Simulink
  cfblk8 : simulink/Discrete/Transfer Fcn First Order  PoleZ=0.95  ICPrevOutput=0.0  DoSatur=off
      settings: SourceProductName=Simulink
  cfblk9 : Delay  DelayLengthSource=Input port
      settings: InputPortMap=u0,p1
  cyemi_{436..445} (10 alike) : DataTypeConversion  OutDataTypeStr=double
  cfblk2 : Outport
  cfblk10 : Outport  Port=2
  wires:
  cfblk1/1 -> cyemi_437/1, cyemi_438/1
  cfblk8/1 -> cfblk2/1
  cfblk5/1 -> cfblk10/1, cyemi_443/1
  cyemi_436/1 -> cfblk11/1
  cfblk9/1 -> cyemi_436/1
  cyemi_437/1 -> cfblk3/1
  cyemi_438/1 -> cfblk4/1
  cyemi_439/1 -> cfblk5/1
  cfblk4/1 -> cyemi_439/1
  cyemi_440/1 -> cfblk6/1
  cfblk11/1 -> cyemi_440/1
  cyemi_441/1 -> cfblk6/2
  cfblk7/1 -> cyemi_441/1
  cyemi_442/1 -> cfblk7/1
  cfblk3/1 -> cyemi_442/1
  cyemi_443/1 -> cfblk8/1
  cyemi_444/1 -> cfblk9/1
  cfblk6/1 -> cyemi_444/1, cyemi_445/1
  cyemi_445/1 -> cfblk9/2

== system sampleModel7127_pp_difftest/cfblk200 ==
  cfblk1 : Inport
  cfblk7 : Inport  Port=2
  Action Port : ActionPort  ActionType=else
  cfblk3 : DiscreteFilter
  cfblk4 : DiscreteFir
  cfblk5 : DiscreteZeroPole  Poles=[0 0.5]  Gain=1  SampleTime=-1
  cfblk6 : Delay
  cfblk9 : Delay
  cyemi_{450..454} (5 alike) : DataTypeConversion  OutDataTypeStr=double
  cfblk2 : Outport
  cfblk8 : Outport  Port=2
  wires:
  cfblk7/1 -> cfblk8/1
  cfblk1/1 -> cfblk2/1
  cyemi_450/1 -> cfblk3/1
  cfblk9/1 -> cyemi_450/1
  cyemi_451/1 -> cfblk4/1
  cfblk6/1 -> cyemi_451/1
  cyemi_452/1 -> cfblk5/1
  cfblk4/1 -> cyemi_452/1
  cyemi_453/1 -> cfblk6/1
  cfblk3/1 -> cyemi_453/1
  cyemi_454/1 -> cfblk9/1
  cfblk5/1 -> cyemi_454/1

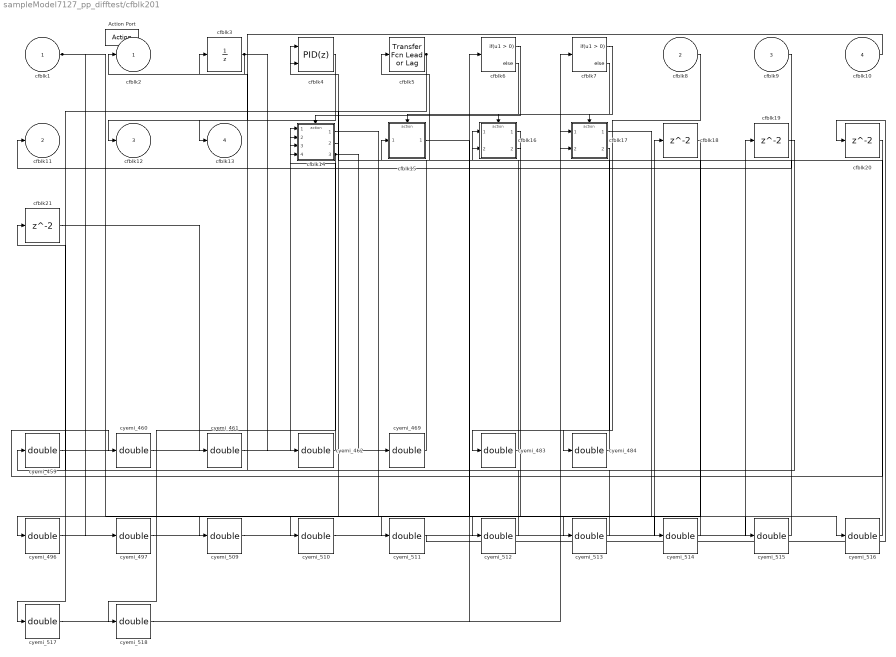
== system sampleModel7127_pp_difftest/cfblk201 ==
  cfblk1 : Inport
  cfblk8 : Inport  Port=2
  cfblk9 : Inport  Port=3
  cfblk10 : Inport  Port=4
  Action Port : ActionPort  ActionType=then
  cfblk14 : Subsystem  TreatAsAtomicUnit=on
  cfblk15 : Subsystem  TreatAsAtomicUnit=on
  cfblk16 : Subsystem  TreatAsAtomicUnit=on
  cfblk17 : Subsystem  TreatAsAtomicUnit=on
  cfblk{18..21} (4 alike) : Delay
  cfblk3 : UnitDelay  SampleTime=-1
  cfblk4 : simulink/Continuous/PID Controller (2DOF)  Controller=PID  TimeDomain=Discrete-time  SampleTime=-1  IntegratorMethod=Forward Euler  FilterMethod=Forward Euler  Form=Parallel  UseFilter=on  ControllerParametersSource=internal  P=1  I=1  D=0  N=100  b=1  c=1  InitialConditionSource=internal  InitialConditionForIntegrator=0  InitialConditionForFilter=0  ExternalReset=none  LimitOutput=off  UpperSaturationLimit=inf  LowerSaturationLimit=-inf  LinearizeAsGain=off  AntiWindupMode=none  Kb=1  TrackingMode=off  Kt=1  PParamMin=[]  PParamMax=[]  IParamMin=[]  IParamMax=[]  DParamMin=[]  DParamMax=[]  NParamMin=[]  NParamMax=[]  bParamMin=[]  bParamMax=[]  cParamMin=[]  cParamMax=[]  KbParamMin=[]  KbParamMax=[]  KtParamMin=[]  KtParamMax=[]  POutMin=[]  POutMax=[]  IOutMin=[]  IOutMax=[]  DOutMin=[]  DOutMax=[]  NOutMin=[]  NOutMax=[]  bOutMin=[]  bOutMax=[]  cOutMin=[]  cOutMax=[]  KbOutMin=[]  KbOutMax=[]  KtOutMin=[]  KtOutMax=[]  IntegratorOutMin=[]  IntegratorOutMax=[]  FilterOutMin=[]  FilterOutMax=[]  SumOutMin=[]  SumOutMax=[]  Sum1OutMin=[]  Sum1OutMax=[]  Sum2OutMin=[]  Sum2OutMax=[]  Sum3OutMin=[]  Sum3OutMax=[]  SumI1OutMin=[]  SumI1OutMax=[]  SumI2OutMin=[]  SumI2OutMax=[]  SumI3OutMin=[]  SumI3OutMax=[]  SumDOutMin=[]  SumDOutMax=[]  SaturationOutMin=[]  SaturationOutMax=[]  IntegratorContinuousStateAttributes=''  IntegratorStateMustResolveToSignalObject=off  IntegratorRTWStateStorageClass=Auto  FilterContinuousStateAttributes=''  FilterStateMustResolveToSignalObject=off  FilterRTWStateStorageClass=Auto  DifferentiatorICPrevScaledInput=0  DifferentiatorOutMin=[]  DifferentiatorOutMax=[]  FilterDiffOutCoefMin=[]  FilterDiffOutCoefMax=[]  SumDenOutMin=[]  SumDenOutMax=[]  SumNumOutMin=[]  SumNumOutMax=[]  ReciprocalOutMin=[]  ReciprocalOutMax=[]  DivideOutMin=[]  DivideOutMax=[]  TunerSelectOption=Transfer Function Based (PID Tuner App)
  cfblk5 : simulink/Discrete/Transfer Fcn Lead or Lag  PoleZ=0.95  ZeroZ=0.75  ICPrevOutput=0.0  ICPrevInput=0.0  DoSatur=off
      settings: SourceProductName=Simulink  SourceProductBaseCode=SL
  cfblk6 : If  SampleTime=1
  cfblk7 : If  SampleTime=1
  cyemi_{459..462,469,483..484,496..497,509..518} (19 alike) : DataTypeConversion  OutDataTypeStr=double
  cfblk2 : Outport
  cfblk11 : Outport  Port=2
  cfblk12 : Outport  Port=3
  cfblk13 : Outport  Port=4
  wires:
  cfblk3/1 -> cfblk2/1, cyemi_462/1
  cfblk1/1 -> cyemi_497/1, cyemi_513/1
  cfblk10/1 -> cfblk13/1
  cfblk14/3(cfblk11) -> cyemi_469/1, cyemi_518/1
  cfblk4/1 -> cfblk12/1
  cfblk5/1 -> cyemi_496/1, cyemi_510/1
  cfblk9/1 -> cfblk11/1
  cfblk6/1 -> cfblk14/Action
  cfblk6/2 -> cfblk15/Action
  cfblk7/1 -> cfblk16/Action
  cfblk7/2 -> cfblk17/Action
  cyemi_459/1 -> cfblk14/1(cfblk1)
  cfblk19/1 -> cyemi_459/1
  cyemi_460/1 -> cfblk14/2(cfblk7)
  cfblk20/1 -> cyemi_460/1
  cyemi_461/1 -> cfblk14/3(cfblk8)
  cfblk21/1 -> cyemi_461/1
  cyemi_462/1 -> cfblk14/4(cfblk9)
  cyemi_469/1 -> cfblk15/1(cfblk1)
  cyemi_483/1 -> cfblk16/1(cfblk1)
  cfblk17/2(cfblk13) -> cyemi_483/1
  cyemi_484/1 -> cfblk16/2(cfblk11)
  cfblk8/1 -> cyemi_484/1
  cyemi_496/1 -> cfblk17/1(cfblk1)
  cyemi_497/1 -> cfblk17/2(cfblk12)
  cyemi_509/1 -> cfblk18/1
  cfblk14/2(cfblk10) -> cyemi_509/1
  cyemi_510/1 -> cfblk19/1
  cyemi_511/1 -> cfblk20/1
  cfblk16/1(cfblk2) -> cyemi_511/1
  cyemi_512/1 -> cfblk21/1
  cfblk16/2(cfblk12) -> cyemi_512/1
  cyemi_513/1 -> cfblk3/1
  cyemi_514/1 -> cfblk4/1
  cfblk14/1(cfblk2) -> cyemi_514/1
  cyemi_515/1 -> cfblk4/2
  cfblk17/1(cfblk2) -> cyemi_515/1
  cyemi_516/1 -> cfblk5/1
  cfblk15/1(cfblk2) -> cyemi_516/1
  cyemi_517/1 -> cfblk6/1
  cfblk18/1 -> cyemi_517/1
  cyemi_518/1 -> cfblk7/1

== system sampleModel7127_pp_difftest/cfblk202 ==
  cfblk1 : Inport
  cfblk11 : Inport  Port=2
  Action Port : ActionPort  ActionType=else
  cfblk10 : simulink/Discrete/Tapped Delay  vinit=0.0  samptime=-1  NumDelays=1  DelayOrder=Oldest  includeCurrent=off
  cfblk3 : UnitDelay  SampleTime=-1
  cfblk4 : UnitDelay  SampleTime=-1
  cfblk5 : simulink/Discrete/Transfer Fcn Real Zero  ZeroZ=0.75  ICPrevInput=0.0  DoSatur=off
      settings: SourceProductName=Simulink  SourceProductBaseCode=SL
  cfblk6 : DiscreteStateSpace  SampleTime=-1
  cfblk7 : DiscreteTransferFcn
  cfblk8 : Delay  ShowEnablePort=on
      settings: InputPortMap=u0,e6
  cfblk9 : simulink/Discrete/Transfer Fcn First Order  PoleZ=0.95  ICPrevOutput=0.0  DoSatur=off
      settings: SourceProductName=Simulink
  cyemi_{521..529} (9 alike) : DataTypeConversion  OutDataTypeStr=double
  cfblk2 : Outport
  cfblk12 : Outport  Port=2
  cfblk13 : Outport  Port=3
  wires:
  cfblk4/1 -> cfblk2/1
  cfblk10/1 -> cyemi_523/1, cyemi_528/1, cyemi_529/1
  cfblk9/1 -> cfblk13/1
  cfblk8/1 -> cfblk12/1
  cyemi_521/1 -> cfblk10/1
  cfblk5/1 -> cyemi_521/1
  cyemi_522/1 -> cfblk3/1
  cfblk7/1 -> cyemi_522/1
  cyemi_523/1 -> cfblk4/1
  cyemi_524/1 -> cfblk5/1
  cfblk11/1 -> cyemi_524/1
  cyemi_525/1 -> cfblk6/1
  cfblk3/1 -> cyemi_525/1
  cyemi_526/1 -> cfblk7/1
  cfblk1/1 -> cyemi_526/1
  cyemi_527/1 -> cfblk8/1
  cfblk6/1 -> cyemi_527/1
  cyemi_528/1 -> cfblk8/2
  cyemi_529/1 -> cfblk9/1

== system sampleModel7127_pp_difftest/cfblk203 ==
  cfblk1 : Inport
  Action Port : ActionPort  ActionType=then
  cfblk11 : Delay
  cfblk12 : Delay
  cfblk13 : DataTypeConversion  OutDataTypeStr=uint32
  cfblk{14..17} (4 alike) : DataTypeConversion  OutDataTypeStr=double
  cfblk3 : simulink/Discrete/Transfer Fcn Real Zero  ZeroZ=0.75  ICPrevInput=0.0  DoSatur=off
      settings: SourceProductName=Simulink  SourceProductBaseCode=SL
  cfblk4 : simulink/Continuous/PID Controller (2DOF)  Controller=PID  TimeDomain=Discrete-time  SampleTime=-1  IntegratorMethod=Forward Euler  FilterMethod=Forward Euler  Form=Parallel  UseFilter=on  ControllerParametersSource=internal  P=1  I=1  D=0  N=100  b=1  c=1  InitialConditionSource=internal  InitialConditionForIntegrator=0  InitialConditionForFilter=0  ExternalReset=none  LimitOutput=off  UpperSaturationLimit=inf  LowerSaturationLimit=-inf  LinearizeAsGain=off  AntiWindupMode=none  Kb=1  TrackingMode=off  Kt=1  PParamMin=[]  PParamMax=[]  IParamMin=[]  IParamMax=[]  DParamMin=[]  DParamMax=[]  NParamMin=[]  NParamMax=[]  bParamMin=[]  bParamMax=[]  cParamMin=[]  cParamMax=[]  KbParamMin=[]  KbParamMax=[]  KtParamMin=[]  KtParamMax=[]  POutMin=[]  POutMax=[]  IOutMin=[]  IOutMax=[]  DOutMin=[]  DOutMax=[]  NOutMin=[]  NOutMax=[]  bOutMin=[]  bOutMax=[]  cOutMin=[]  cOutMax=[]  KbOutMin=[]  KbOutMax=[]  KtOutMin=[]  KtOutMax=[]  IntegratorOutMin=[]  IntegratorOutMax=[]  FilterOutMin=[]  FilterOutMax=[]  SumOutMin=[]  SumOutMax=[]  Sum1OutMin=[]  Sum1OutMax=[]  Sum2OutMin=[]  Sum2OutMax=[]  Sum3OutMin=[]  Sum3OutMax=[]  SumI1OutMin=[]  SumI1OutMax=[]  SumI2OutMin=[]  SumI2OutMax=[]  SumI3OutMin=[]  SumI3OutMax=[]  SumDOutMin=[]  SumDOutMax=[]  SaturationOutMin=[]  SaturationOutMax=[]  IntegratorContinuousStateAttributes=''  IntegratorStateMustResolveToSignalObject=off  IntegratorRTWStateStorageClass=Auto  FilterContinuousStateAttributes=''  FilterStateMustResolveToSignalObject=off  FilterRTWStateStorageClass=Auto  DifferentiatorICPrevScaledInput=0  DifferentiatorOutMin=[]  DifferentiatorOutMax=[]  FilterDiffOutCoefMin=[]  FilterDiffOutCoefMax=[]  SumDenOutMin=[]  SumDenOutMax=[]  SumNumOutMin=[]  SumNumOutMax=[]  ReciprocalOutMin=[]  ReciprocalOutMax=[]  DivideOutMin=[]  DivideOutMax=[]  TunerSelectOption=Transfer Function Based (PID Tuner App)
  cfblk5 : simulink/Discrete/Transfer Fcn Lead or Lag  PoleZ=0.95  ZeroZ=0.75  ICPrevOutput=0.0  ICPrevInput=0.0  DoSatur=off
      settings: SourceProductName=Simulink  SourceProductBaseCode=SL
  cfblk6 : DiscreteFir
  cfblk7 : Delay
  cyemi_{531..532,536..538,542..543} (7 alike) : DataTypeConversion  OutDataTypeStr=uint32
  cyemi_{533..535,539..541} (6 alike) : DataTypeConversion  OutDataTypeStr=double
  cfblk2 : Outport
  cfblk8 : Outport  Port=2
  cfblk9 : Outport  Port=3
  cfblk10 : Outport  Port=4
  wires:
  cfblk1/1 -> cfblk9/1
  cfblk6/1 -> cfblk8/1
  cfblk3/1 -> cyemi_536/1, cyemi_543/1
  cfblk13/1 -> cfblk10/1, cfblk2/1, cyemi_531/1, cyemi_532/1
  cyemi_531/1 -> cfblk11/1
  cyemi_532/1 -> cfblk12/1
  cyemi_533/1 -> cfblk13/1
  cfblk5/1 -> cyemi_533/1
  cyemi_534/1 -> cfblk14/1
  cfblk15/1 -> cyemi_534/1
  cyemi_535/1 -> cfblk15/1
  cfblk4/1 -> cyemi_535/1
  cyemi_536/1 -> cfblk16/1
  cyemi_537/1 -> cfblk17/1
  cfblk11/1 -> cyemi_537/1
  cyemi_538/1 -> cfblk3/1
  cfblk12/1 -> cyemi_538/1
  cyemi_539/1 -> cfblk4/1
  cfblk16/1 -> cyemi_539/1
  cyemi_540/1 -> cfblk4/2
  cfblk17/1 -> cyemi_540/1
  cyemi_541/1 -> cfblk5/1
  cfblk14/1 -> cyemi_541/1
  cyemi_542/1 -> cfblk6/1
  cfblk7/1 -> cyemi_542/1
  cyemi_543/1 -> cfblk7/1

== system sampleModel7127_pp_difftest/cfblk204 ==
  cfblk1 : Inport
  Action Port : ActionPort  ActionType=else
  cfblk11 : Delay
  cfblk3 : Delay  ShowEnablePort=on
      settings: InputPortMap=u0,e6
  cfblk4 : Delay  ShowEnablePort=on
      settings: InputPortMap=u0,e6
  cfblk5 : simulink/Discrete/Transfer Fcn First Order  PoleZ=0.95  ICPrevOutput=0.0  DoSatur=off
      settings: SourceProductName=Simulink
  cfblk6 : UnitDelay  SampleTime=-1
  cfblk7 : DiscreteZeroPole  Poles=[0 0.5]  Gain=1  SampleTime=-1
  cfblk8 : DiscreteStateSpace  SampleTime=-1
  cyemi_{545..553} (9 alike) : DataTypeConversion  OutDataTypeStr=double
  cfblk2 : Outport
  cfblk9 : Outport  Port=2
  cfblk10 : Outport  Port=3
  wires:
  cfblk8/1 -> cfblk9/1
  cfblk4/1 -> cyemi_550/1, cyemi_552/1
  cfblk6/1 -> cfblk2/1, cyemi_553/1
  cfblk5/1 -> cfblk10/1, cyemi_545/1
  cyemi_545/1 -> cfblk11/1
  cyemi_546/1 -> cfblk3/1
  cfblk7/1 -> cyemi_546/1, cyemi_547/1
  cyemi_547/1 -> cfblk3/2
  cyemi_548/1 -> cfblk4/1
  cfblk1/1 -> cyemi_548/1
  cyemi_549/1 -> cfblk4/2
  cfblk11/1 -> cyemi_549/1
  cyemi_550/1 -> cfblk5/1
  cyemi_551/1 -> cfblk6/1
  cfblk3/1 -> cyemi_551/1
  cyemi_552/1 -> cfblk7/1
  cyemi_553/1 -> cfblk8/1

== system sampleModel7127_pp_difftest/cfblk205 ==
  cfblk1 : Inport
  cfblk8 : Inport  Port=2
  Action Port : ActionPort  ActionType=then
  cfblk10 : Delay
  cfblk3 : DiscreteStateSpace  SampleTime=-1
  cfblk4 : DiscreteIntegrator  SampleTime=-1  OutDataTypeStr=double  ICPrevOutput=DiscIntNeverNeededParam  ICPrevScaledInput=DiscIntNeverNeededParam
  cfblk5 : Delay
  cfblk6 : UnitDelay  SampleTime=-1
  cfblk7 : simulink/Continuous/PID Controller (2DOF)  Controller=PID  TimeDomain=Discrete-time  SampleTime=-1  IntegratorMethod=Forward Euler  FilterMethod=Forward Euler  Form=Parallel  UseFilter=on  ControllerParametersSource=internal  P=1  I=1  D=0  N=100  b=1  c=1  InitialConditionSource=internal  InitialConditionForIntegrator=0  InitialConditionForFilter=0  ExternalReset=none  LimitOutput=off  UpperSaturationLimit=inf  LowerSaturationLimit=-inf  LinearizeAsGain=off  AntiWindupMode=none  Kb=1  TrackingMode=off  Kt=1  PParamMin=[]  PParamMax=[]  IParamMin=[]  IParamMax=[]  DParamMin=[]  DParamMax=[]  NParamMin=[]  NParamMax=[]  bParamMin=[]  bParamMax=[]  cParamMin=[]  cParamMax=[]  KbParamMin=[]  KbParamMax=[]  KtParamMin=[]  KtParamMax=[]  POutMin=[]  POutMax=[]  IOutMin=[]  IOutMax=[]  DOutMin=[]  DOutMax=[]  NOutMin=[]  NOutMax=[]  bOutMin=[]  bOutMax=[]  cOutMin=[]  cOutMax=[]  KbOutMin=[]  KbOutMax=[]  KtOutMin=[]  KtOutMax=[]  IntegratorOutMin=[]  IntegratorOutMax=[]  FilterOutMin=[]  FilterOutMax=[]  SumOutMin=[]  SumOutMax=[]  Sum1OutMin=[]  Sum1OutMax=[]  Sum2OutMin=[]  Sum2OutMax=[]  Sum3OutMin=[]  Sum3OutMax=[]  SumI1OutMin=[]  SumI1OutMax=[]  SumI2OutMin=[]  SumI2OutMax=[]  SumI3OutMin=[]  SumI3OutMax=[]  SumDOutMin=[]  SumDOutMax=[]  SaturationOutMin=[]  SaturationOutMax=[]  IntegratorContinuousStateAttributes=''  IntegratorStateMustResolveToSignalObject=off  IntegratorRTWStateStorageClass=Auto  FilterContinuousStateAttributes=''  FilterStateMustResolveToSignalObject=off  FilterRTWStateStorageClass=Auto  DifferentiatorICPrevScaledInput=0  DifferentiatorOutMin=[]  DifferentiatorOutMax=[]  FilterDiffOutCoefMin=[]  FilterDiffOutCoefMax=[]  SumDenOutMin=[]  SumDenOutMax=[]  SumNumOutMin=[]  SumNumOutMax=[]  ReciprocalOutMin=[]  ReciprocalOutMax=[]  DivideOutMin=[]  DivideOutMax=[]  TunerSelectOption=Transfer Function Based (PID Tuner App)
  cyemi_{556..562} (7 alike) : DataTypeConversion  OutDataTypeStr=double
  cfblk2 : Outport
  cfblk9 : Outport  Port=2
  wires:
  cfblk3/1 -> cfblk2/1
  cfblk6/1 -> cfblk9/1, cyemi_556/1
  cyemi_556/1 -> cfblk10/1
  cyemi_557/1 -> cfblk3/1
  cfblk5/1 -> cyemi_557/1
  cyemi_558/1 -> cfblk4/1
  cfblk10/1 -> cyemi_558/1
  cyemi_559/1 -> cfblk5/1
  cfblk1/1 -> cyemi_559/1
  cyemi_560/1 -> cfblk6/1
  cfblk7/1 -> cyemi_560/1
  cyemi_561/1 -> cfblk7/1
  cfblk8/1 -> cyemi_561/1
  cyemi_562/1 -> cfblk7/2
  cfblk4/1 -> cyemi_562/1
